simulink model "ROS2ValetBehavioralPlannerExample"  (R2022b)
settings: Solver=FixedStepAuto  StartTime=0.0  StopTime=inf  RelTol=1e-3
model workspace (MAT data in the model file):
  SL_ROS_VariableLengthArrays_MaxSizes.CommonInfo.ArrayTruncateAction = 'EmitWarning'
  SL_ROS_VariableLengthArrays_MaxSizes.MsgTypeMap = containers.Map
  SL_ROS_VariableLengthArrays_MaxSizes.MsgTypeMap.serialization.keys = {'std_msgs/Float64MultiArray'}
  SL_ROS_VariableLengthArrays_MaxSizes.MsgTypeMap.serialization.values{1}.PropertyName = 'data'
  SL_ROS_VariableLengthArrays_MaxSizes.MsgTypeMap.serialization.values{1}.DataType = 'double'
  SL_ROS_VariableLengthArrays_MaxSizes.MsgTypeMap.serialization.values{1}.MaxLength = 1500
  SL_ROS_VariableLengthArrays_MaxSizes.MsgTypeMap.serialization.uniformity = 0
  SL_ROS_VariableLengthArrays_MaxSizes.MsgTypeMap.serialization.keyType = 'char'
  SL_ROS_VariableLengthArrays_MaxSizes.MsgTypeMap.serialization.valueType = 'any'
values from neighbouring files (symbols this model uses):
  routePlan = table2struct(routePlan)    [ExampleHelperROSValetBehavioralPlanner.m]
undefined symbols (not defined in the file or in its folder): data, data_SL_Info, theta, x, y
libraries: ros2lib x11
settings Model: Creator=The MathWorks, Inc.  LastModifiedBy=The MathWorks, Inc.
settings SolverCC: AlgebraicLoopSolver=TrustRegion
settings OptimizationCC: EnhancedBackFolding=on  PassReuseOutputArgsAs=Individual arguments  ZeroExternalMemoryAtStartup=off  ZeroInternalMemoryAtStartup=off  MaxStackSize=64  OptimizeBlockOrder=speed  DifferentSizesBufferReuse=on  OptimizationCustomize=off  EfficientTunableParamExpr=on
settings DebuggingCC: ParameterTunabilityLossMsg=error  UnconnectedInputMsg=warning  UnconnectedOutputMsg=warning  UnconnectedLineMsg=warning  SymbolicDimsDataTypeCodeGenerationDiagnostic=none  SFMachineParentedDataDiag=warning
settings ModelReferenceCC: EnableRefExpFcnMdlSchedulingChecks=on
settings SFSimCC: MATLABDynamicMemAlloc=off  SimTargetLang=C++
settings RTWCC: Description=Embedded Coder  SystemTargetFile=ert.tlc  HardwareBoard=Robot Operating System 2 (ROS 2)  TLCOptions=-aInlineSetEventsForThisBaseRateFcn=TLC_FALSE -aSuppressMultiTaskScheduler=TLC_FALSE -aRateBasedStepFcn=1  TemplateMakefile=ert_default_tmf  GenerateReport=on  Toolchain=Colcon Tools  IncludeHyperlinkInReport=on  LaunchReport=on  TargetLang=C++  GenerateTraceInfo=on  GenerateTraceReport=on  GenerateTraceReportSl=on  GenerateTraceReportSf=on  GenerateTraceReportEml=on
settings CodeAppCC: ForceParamTrailComments=on  IgnoreCustomStorageClasses=off  OperatorAnnotations=on  SimulinkDataObjDesc=on  SFDataObjDesc=on  InsertBlockDesc=on
settings ERTTargetCC: CodeInterfacePackaging=C++ class  RootIOFormat=Structure reference

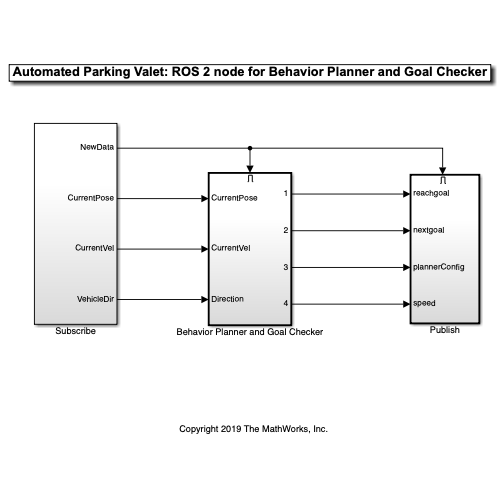
[thumbnail: Simulink's stored preview of the top-level diagram]
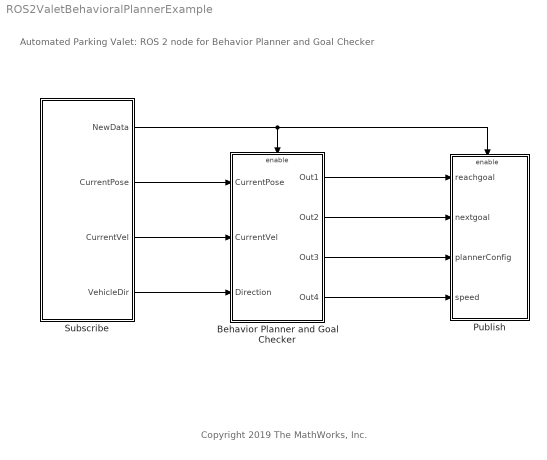
== system ROS2ValetBehavioralPlannerExample ==
  note: Automated Parking Valet: ROS 2 node for Behavior Planner and Goal Checker
  note: Copyright 2019 The MathWorks, Inc.
  Behavior Planner and Goal Checker : Subsystem
  Publish : Subsystem
  Subscribe : Subsystem
  wires:
  Subscribe/2(CurrentPose) -> Behavior Planner and Goal Checker/1(CurrentPose)
  Subscribe/3(CurrentVel) -> Behavior Planner and Goal Checker/2(CurrentVel)
  Subscribe/4(VehicleDir) -> Behavior Planner and Goal Checker/3(Direction)
  Subscribe/1(NewData) -> Behavior Planner and Goal Checker/Enable, Publish/Enable
  Behavior Planner and Goal Checker/1(Out1) -> Publish/1(reachgoal)
  Behavior Planner and Goal Checker/2(Out2) -> Publish/2(nextgoal)
  Behavior Planner and Goal Checker/3(Out3) -> Publish/3(plannerConfig)
  Behavior Planner and Goal Checker/4(Out4) -> Publish/4(speed)

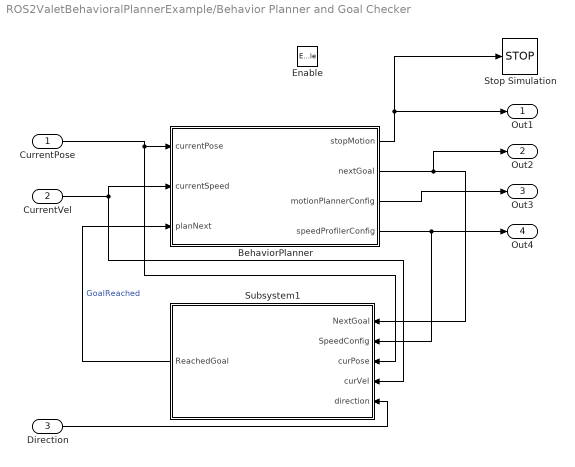
== system ROS2ValetBehavioralPlannerExample/Behavior Planner and Goal Checker ==
  CurrentPose : Inport
  CurrentVel : Inport  Port=2
  Direction : Inport  Port=3
  Enable : EnablePort  PropagateVarSize=During execution
  BehaviorPlanner : MATLAB Function  TreatAsAtomicUnit=on  mask{RoutePlan=routePlan, StartSpeed=0}
      mask prompts: RoutePlan "Route plan:"; StartSpeed "Initial vehicle speed  [m/s]:"
      mask init:
      | validateattributes(RoutePlan, {'table'}, {'ncols', 3});
      | validateattributes(StartSpeed, {'double'}, {'scalar','nonnegative'})
      | 
      | routePlanStruct   = table2struct(RoutePlan);
      | startPose         = routePlanStruct(1).StartPose;
  Stop Simulation : Stop
  Subsystem1 : Subsystem  TreatAsAtomicUnit=on  SystemSampleTime=0.1
      settings: MinAlgLoopOccurrences=on
      mask Display:
      | disp(['Helper' char(10) 'Goal' char(10) 'Checker']);
      | port_label('input',1,'NextGoal');
      | port_label('input',2,'SpeedConfig');
      | port_label('input',3,'CurPose');
      | port_label('input',4,'CurVel');
      | port_label('input',5,'Direction');
      | port_label('output',1,'GoalReached');
  Out1 : Outport
  Out2 : Outport  Port=2
  Out3 : Outport  Port=3
  Out4 : Outport  Port=4
  wires:
  BehaviorPlanner/4(speedProfilerConfig) -> Out4/1, Subsystem1/2(SpeedConfig)
  BehaviorPlanner/1(stopMotion) -> Stop Simulation/1, Out1/1
  CurrentVel/1 -> BehaviorPlanner/2(currentSpeed), Subsystem1/4(curVel)
  Direction/1 -> Subsystem1/5(direction)
  BehaviorPlanner/2(nextGoal) -> Out2/1, Subsystem1/1(NextGoal)
  CurrentPose/1 -> Subsystem1/3(curPose), BehaviorPlanner/1(currentPose)
  Subsystem1/1(ReachedGoal) -> BehaviorPlanner/3(planNext)  "GoalReached"
  BehaviorPlanner/3(motionPlannerConfig) -> Out3/1

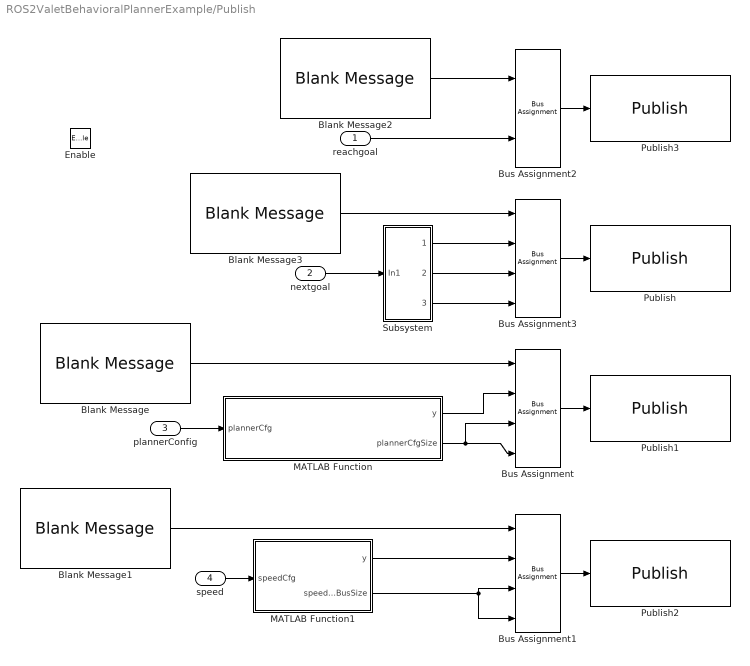
== system ROS2ValetBehavioralPlannerExample/Publish ==
  reachgoal : Inport
  nextgoal : Inport  Port=2
  plannerConfig : Inport  Port=3
  speed : Inport  Port=4
  Enable : EnablePort
  Blank Message : ros2lib/Blank Message  messageClass=Message  entityType=std_msgs/Float64MultiArray  messageType=std_msgs/Float64MultiArray  SampleTime=-1
  Blank Message1 : ros2lib/Blank Message  messageClass=Message  entityType=std_msgs/Float64MultiArray  messageType=std_msgs/Float64MultiArray  SampleTime=-1
  Blank Message2 : ros2lib/Blank Message  messageClass=Message  entityType=std_msgs/Bool  messageType=std_msgs/Bool  SampleTime=-1
  Blank Message3 : ros2lib/Blank Message  messageClass=Message  entityType=geometry_msgs/Pose2D  messageType=geometry_msgs/Pose2D  SampleTime=-1
  Bus Assignment : BusAssignment  AssignedSignals=data,data_SL_Info.CurrentLength,data_SL_Info.ReceivedLength
  Bus Assignment1 : BusAssignment  AssignedSignals=data,data_SL_Info.CurrentLength,data_SL_Info.ReceivedLength
  Bus Assignment2 : BusAssignment  AssignedSignals=data
  Bus Assignment3 : BusAssignment  AssignedSignals=x,y,theta
  MATLAB Function : MATLAB Function  TreatAsAtomicUnit=on
  MATLAB Function1 : MATLAB Function  TreatAsAtomicUnit=on
  Publish : ros2lib/Publish  topicSource=Select from ROS network  topic=/nextgoal  messageType=geometry_msgs/Pose2D  QOSHistory=Keep last  QOSDepth=1  QOSReliability=Reliable  QOSDurability=Volatile
  Publish1 : ros2lib/Publish  topicSource=Specify your own  topic=/plannerConfig  messageType=std_msgs/Float64MultiArray  QOSHistory=Keep last  QOSDepth=1  QOSReliability=Reliable  QOSDurability=Volatile
  Publish2 : ros2lib/Publish  topicSource=Specify your own  topic=/speed  messageType=std_msgs/Float64MultiArray  QOSHistory=Keep last  QOSDepth=1  QOSReliability=Reliable  QOSDurability=Volatile
  Publish3 : ros2lib/Publish  topicSource=Specify your own  topic=/reachgoal  messageType=std_msgs/Bool  QOSHistory=Keep last  QOSDepth=1  QOSReliability=Reliable  QOSDurability=Volatile
  Subsystem : Subsystem
  wires:
  MATLAB Function/1(y) -> Bus Assignment/2
  speed/1 -> MATLAB Function1/1(speedCfg)
  MATLAB Function1/2(speedCfgBusSize) -> Bus Assignment1/4, Bus Assignment1/3
  Subsystem/3(Out3) -> Bus Assignment3/4
  Bus Assignment/1 -> Publish1/1
  Blank Message/1 -> Bus Assignment/1
  MATLAB Function/2(plannerCfgSize) -> Bus Assignment/3, Bus Assignment/4
  MATLAB Function1/1(y) -> Bus Assignment1/2
  Blank Message1/1 -> Bus Assignment1/1
  Bus Assignment3/1 -> Publish/1
  Blank Message3/1 -> Bus Assignment3/1
  Blank Message2/1 -> Bus Assignment2/1
  Bus Assignment2/1 -> Publish3/1
  Bus Assignment1/1 -> Publish2/1
  Subsystem/1(Out1) -> Bus Assignment3/2
  Subsystem/2(Out2) -> Bus Assignment3/3
  reachgoal/1 -> Bus Assignment2/2
  plannerConfig/1 -> MATLAB Function/1(plannerCfg)
  nextgoal/1 -> Subsystem/1(In1)

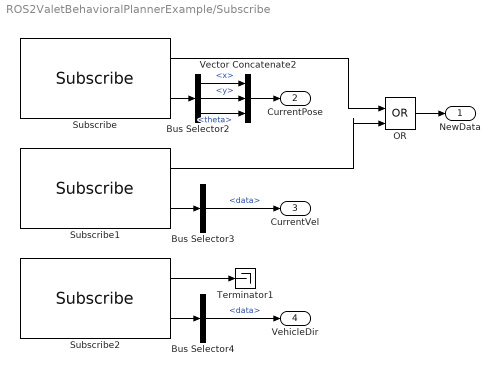
== system ROS2ValetBehavioralPlannerExample/Subscribe ==
  Bus Selector2 : BusSelector  OutputSignals=x,y,theta
  Bus Selector3 : BusSelector  OutputSignals=data
  Bus Selector4 : BusSelector  OutputSignals=data
  OR : Logic  Operator=OR  IconShape=distinctive  AllPortsSameDT=off  OutDataTypeStr=boolean
  Subscribe : ros2lib/Subscribe  topicSource=Select from ROS network  topic=/currentpose  messageType=geometry_msgs/Pose2D  sampleTime=-1  QOSHistory=Keep last  QOSDepth=1  QOSReliability=Reliable  QOSDurability=Volatile
  Subscribe1 : ros2lib/Subscribe  topicSource=Select from ROS network  topic=/currentvel  messageType=std_msgs/Float64  sampleTime=-1  QOSHistory=Keep last  QOSDepth=1  QOSReliability=Reliable  QOSDurability=Volatile
  Subscribe2 : ros2lib/Subscribe  topicSource=Select from ROS network  topic=/vehdir  messageType=std_msgs/Float64  sampleTime=-1  QOSHistory=Keep last  QOSDepth=1  QOSReliability=Reliable  QOSDurability=Volatile
  Terminator1 : Terminator
  Vector Concatenate2 : Concatenate  NumInputs=3
  NewData : Outport  VectorParamsAs1DForOutWhenUnconnected=off
  CurrentPose : Outport  Port=2  VectorParamsAs1DForOutWhenUnconnected=off
  CurrentVel : Outport  Port=3  VectorParamsAs1DForOutWhenUnconnected=off
  VehicleDir : Outport  Port=4  VectorParamsAs1DForOutWhenUnconnected=off
  wires:
  Subscribe1/2 -> Bus Selector3/1
  Subscribe2/2 -> Bus Selector4/1
  Bus Selector2/3 -> Vector Concatenate2/3  "<theta>"
  Bus Selector2/2 -> Vector Concatenate2/2  "<y>"
  Bus Selector2/1 -> Vector Concatenate2/1  "<x>"
  Bus Selector4/1 -> VehicleDir/1  "<data>"
  Bus Selector3/1 -> CurrentVel/1  "<data>"
  Subscribe/2 -> Bus Selector2/1
  Vector Concatenate2/1 -> CurrentPose/1
  Subscribe2/1 -> Terminator1/1
  Subscribe/1 -> OR/1
  Subscribe1/1 -> OR/2
  OR/1 -> NewData/1

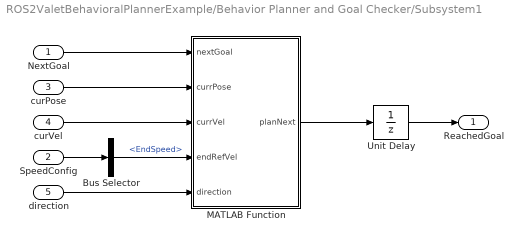
== system ROS2ValetBehavioralPlannerExample/Behavior Planner and Goal Checker/Subsystem1 ==
  NextGoal : Inport
  SpeedConfig : Inport  Port=2
  curPose : Inport  Port=3
  curVel : Inport  Port=4
  direction : Inport  Port=5
  Bus Selector : BusSelector  OutputSignals=EndSpeed
  MATLAB Function : MATLAB Function  TreatAsAtomicUnit=on
  Unit Delay : UnitDelay  SampleTime=-1  HasFrameUpgradeWarning=on
  ReachedGoal : Outport  VectorParamsAs1DForOutWhenUnconnected=off
  wires:
  Bus Selector/1 -> MATLAB Function/4(endRefVel)  "<EndSpeed>"
  Unit Delay/1 -> ReachedGoal/1
  SpeedConfig/1 -> Bus Selector/1
  MATLAB Function/1(planNext) -> Unit Delay/1
  NextGoal/1 -> MATLAB Function/1(nextGoal)
  curPose/1 -> MATLAB Function/2(currPose)
  curVel/1 -> MATLAB Function/3(currVel)
  direction/1 -> MATLAB Function/5(direction)

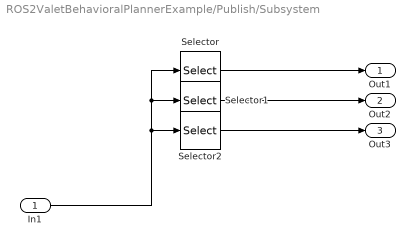
== system ROS2ValetBehavioralPlannerExample/Publish/Subsystem ==
  In1 : Inport
  Selector : Selector  InputPortWidth=3  IndexOptions=Index vector (dialog)  Indices=1  OutputSizes=1
  Selector1 : Selector  InputPortWidth=3  IndexOptions=Index vector (dialog)  Indices=2  OutputSizes=1
  Selector2 : Selector  InputPortWidth=3  IndexOptions=Index vector (dialog)  Indices=3  OutputSizes=1
  Out1 : Outport
  Out2 : Outport  Port=2
  Out3 : Outport  Port=3
  wires:
  In1/1 -> Selector/1, Selector1/1, Selector2/1
  Selector/1 -> Out1/1
  Selector2/1 -> Out3/1
  Selector1/1 -> Out2/1

== matlab function ROS2ValetBehavioralPlannerExample/Publish/MATLAB Function1 ==
  data: speedCfg input Bus: speedConfigBus; y output double size=[1 1500]; speedCfgBusSize output uint32
function [y, speedCfgBusSize] = extractSpeedCfg(speedCfg)
y = zeros(1,1500);
speedCfgBusSize = uint32(3);
y(1:speedCfgBusSize) = [speedCfg.StartSpeed speedCfg.EndSpeed speedCfg.MaxSpeed];

== matlab function ROS2ValetBehavioralPlannerExample/Publish/MATLAB Function ==
  data: plannerCfg input Bus: plannerConfigBus; y output double size=[1 1500]; plannerCfgSize output uint32 size=[1 1]
function [y, plannerCfgSize] = extractPlannerCfg(plannerCfg)
y = zeros(1,1500);
plannerCfgSize = uint32(6);
y(1:plannerCfgSize) = [plannerCfg.ConnectionDistance, plannerCfg.MinIterations, plannerCfg.GoalTolerance, plannerCfg.MinTurningRadius];

== matlab function ROS2ValetBehavioralPlannerExample/Behavior Planner and Goal Checker/Subsystem1/MATLAB Function ==
  data: nextGoal input size=[1 3]; planNext output size=[1 1]; currPose input size=[1 3]; currVel input size=[1 1]; endRefVel input size=[1 1]; direction input
function planNext = goalCheker(nextGoal, currPose, currVel, endRefVel, direction)

planNext = exampleHelperROSValetGoalChecker(nextGoal, currPose, currVel, endRefVel, direction);

== matlab function ROS2ValetBehavioralPlannerExample/Behavior Planner and Goal Checker/BehaviorPlanner ==
  settings: updateMethod=DISCRETE  sampleTime=0.1
  data: stopMotion output; nextGoal output double size=[1 3]; motionPlannerConfig output Bus: plannerConfigBus; speedProfilerConfig output Bus: speedConfigBus; routePlanStruct parameter; currentPose input size=[1 3]; currentSpeed input size=[1 1]; planNext input size=[1 1]; startPose parameter size=[1 3]; StartSpeed parameter
function [stopMotion, nextGoal, motionPlannerConfig, speedProfilerConfig] = ...
    behaviorPlanning(routePlanStruct, currentPose, currentSpeed, planNext, ...
    startPose, StartSpeed)

%behaviorPlanning generate navigation tasks and configurations for the 
%   Motion Planner block and the Trajectory Generator block.

nextGoal     = coder.nullcopy(zeros(1, 3)); %#ok<*NASGU>
stopMotion   = coder.nullcopy(logical(0));  %#ok<*LOGL>

persistent behavioralPlanner
persistent nextGoalPose plannerConfig speedConfig
persistent pose speed

if isempty(behavioralPlanner)
    
    % Initialize pose and speed
    pose  = startPose;
    speed = StartSpeed;
    
    % Initialize planner
    steerLimit = 30;
    behavioralPlanner = ExampleHelperROSValetBehavioralPlanner(routePlanStruct, steerLimit);
    [nextGoalPose, plannerConfig, speedConfig] = requestManeuver( ...
        behavioralPlanner, pose, speed);
end

pose  = currentPose;
speed = currentSpeed;

disTol = 1;
% Plan a new path when reaching the goal
if planNext && ~reachedDestination(behavioralPlanner)
    [nextGoalPose, plannerConfig, speedConfig] = requestManeuver( ...
        behavioralPlanner, pose, speed);
end

% Stop motion when reaching the destination
stopMotion = planNext && reachedDestination(behavioralPlanner) && ...
    norm(pose(1:2) - nextGoalPose(1:2)) < disTol;
    
nextGoal            = nextGoalPose;
motionPlannerConfig.ConnectionDistance = plannerConfig.ConnectionDistance;
motionPlannerConfig.MinIterations = plannerConfig.MinIterations;
motionPlannerConfig.GoalTolerance = plannerConfig.GoalTolerance;
motionPlannerConfig.MinTurningRadius = plannerConfig.MinTurningRadius;
speedProfilerConfig = speedConfig;

end
